simulink model "dpd_pa"  (Simulink 8.7)
settings: Solver=VariableStepDiscrete  StartTime=0.0  StopTime=hepta_dpd_pa_param.endTime  RelTol=1e-3
PreLoadFcn:
  | % Run the setup script when the model is opened
  | setup_dpd_pa;
InitFcn:
  | % Run the setup script again just before the
  | % model is run, so that any updates made
  | % after opening are applied.
  | setup_dpd_pa;
undefined symbols (not defined in the file or in its folder): AdvDSPBChannelOutDisplay, dpoly, dspba_ChannelInVis, dspba_ChannelOutVis, dspba_internal_get_channel_ports, evalAionMaskParam, hepta_dpd_pa_param, latency, value
libraries: DSPBAPrim x159, DSPBABase x6, DSPBAAvalonST x2, DSPBAUtilities x1
(part 2 of 2)

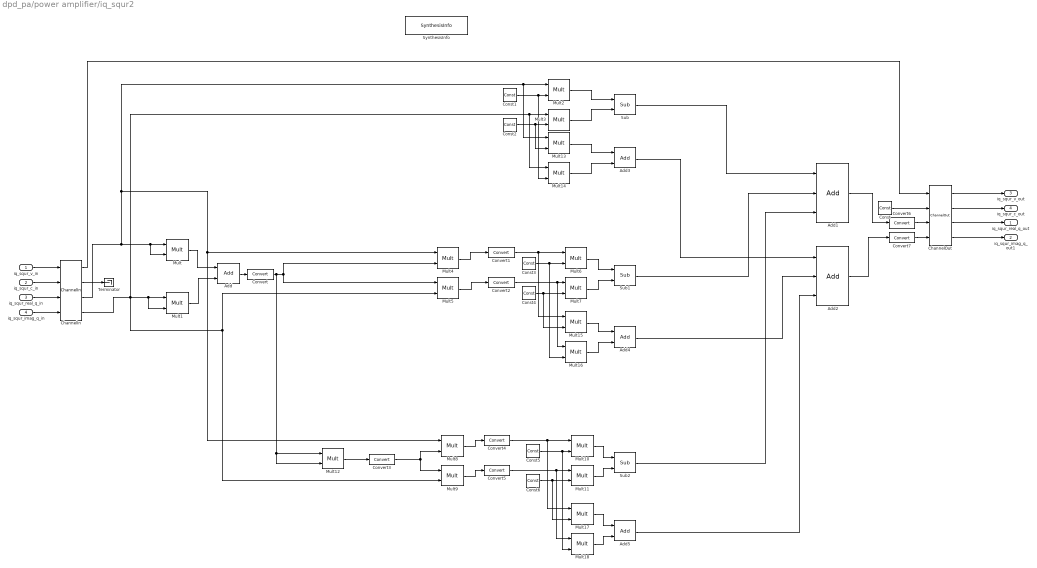
== system dpd_pa/power amplifier/iq_squr2 ==
  iq_squr_v_in : Inport
  iq_squr_c_in : Inport  Port=2
  iq_squr_real_q_in : Inport  Port=3
  iq_squr_imag_q_in : Inport  Port=4
  Add{,3..5} (4 alike) : DSPBAPrim/Add  primtype=add  nInputs=evalAionMaskParam(gcb,'value',1)  nOutputs=1  omode=Inherit via internal rule with word growth  otype=sfix(16)  scale=2^-15  rndmethod=Unbiased  factor=1  satmethod=Symmetric  shift_vec=[0 1 2 -1]  value=2  inPortNames=[' '; ' ';]  outPortNames=[' ']  dspbaimage=dspba_prim.jpg  text=fprintf('+');  style=Optimised  visibilities=1032+2^17+2^18+2^19  genFPC=off  floatRounding=correct  advOptions=[]  version=20130821
  Add1 : DSPBAPrim/Add  primtype=add  nInputs=evalAionMaskParam(gcb,'value',1)  nOutputs=1  omode=Inherit via internal rule with word growth  otype=sfix(16)  scale=2^-15  rndmethod=Unbiased  factor=1  satmethod=Symmetric  shift_vec=[0 1 2 -1]  value=3  inPortNames=[' '; ' ';]  outPortNames=[' ']  dspbaimage=dspba_prim.jpg  text=fprintf('+');  style=Optimised  visibilities=1032+2^17+2^18+2^19  genFPC=off  floatRounding=correct  advOptions=[]  version=20130821
  Add2 : DSPBAPrim/Add  primtype=add  nInputs=evalAionMaskParam(gcb,'value',1)  nOutputs=1  omode=Inherit via internal rule with word growth  otype=sfix(16)  scale=2^-15  rndmethod=Unbiased  factor=1  satmethod=Symmetric  shift_vec=[0 1 2 -1]  value=3  inPortNames=[' '; ' ';]  outPortNames=[' ']  dspbaimage=dspba_prim.jpg  text=fprintf('+');  style=Optimised  visibilities=1032+2^17+2^18+2^19  genFPC=off  floatRounding=correct  advOptions=[]  version=20130821
  ChannelIn : DSPBAPrim/ChannelIn  primtype=channelin  nInputs=dspba_internal_get_channel_ports(gcb)  nOutputs=dspba_internal_get_channel_ports(gcb)  omode=Inherit via internal rule  otype=sfix(16)  scale=2^-15  rndmethod=Unbiased  factor=1  satmethod=Symmetric  shift_vec=[0 1 2 -1]  value=2  inPortNames=['v'; 'c'; '0'; '1'; '2'; '3'; '4'; '5'; '6'; '7'; '8'; '9'; 'A'; 'B'; 'D'; 'E'; 'F'; 'G'; 'H'; 'I'; 'J'; 'K'; 'L'; 'M'; 'N'; 'O'; 'P'; 'Q'; 'R'; 'S'; 'T'; 'U'; 'W'; 'X'; 'Y'; 'Z']  outPortNames=['v'; 'c'; '0'; '1'; '2'; '3'; '4'; '5'; '6'; '7'; '8'; '9'; 'A'; 'B'; 'D'; 'E'; 'F'; 'G'; 'H'; 'I'; 'J'; 'K'; 'L'; 'M'; 'N'; 'O'; 'P'; 'Q'; 'R'; 'S'; 'T'; 'U'; 'W'; 'X'; 'Y'; 'Z']  dspbaimage=dspba_prim.jpg  text=fprintf('In');  style=Optimised  dataSignals=2  foldingEnabled=off  channels=1  sampleRate=200  packetBeginPresent=off  packetBeginEnabled=off  visibilities=dspba_ChannelInVis(gcb)  latencyCorrection=0  version=20141013
  ChannelOut : DSPBAPrim/ChannelOut  primtype=channelout  nInputs=dspba_internal_get_channel_ports(gcb)  nOutputs=dspba_internal_get_channel_ports(gcb)  omode=Inherit via internal rule  otype=sfix(16)  scale=2^-15  rndmethod=Unbiased  factor=1  satmethod=Symmetric  shift_vec=[0 1 2 -1]  value=2  inPortNames=['v'; 'c'; '0'; '1'; '2'; '3'; '4'; '5'; '6'; '7'; '8'; '9'; 'A'; 'B'; 'D'; 'E'; 'F'; 'G'; 'H'; 'I'; 'J'; 'K'; 'L'; 'M'; 'N'; 'O'; 'P'; 'Q'; 'R'; 'S'; 'T'; 'U'; 'W'; 'X'; 'Y'; 'Z']  outPortNames=['v'; 'c'; '0'; '1'; '2'; '3'; '4'; '5'; '6'; '7'; '8'; '9'; 'A'; 'B'; 'D'; 'E'; 'F'; 'G'; 'H'; 'I'; 'J'; 'K'; 'L'; 'M'; 'N'; 'O'; 'P'; 'Q'; 'R'; 'S'; 'T'; 'U'; 'W'; 'X'; 'Y'; 'Z']  dspbaimage=dspba_prim.jpg  text=fprintf('Out%s', AdvDSPBChannelOutDisplay(latency));  style=Optimised  dataSignals=2  foldingEnabled=off  channels=1  sampleRate=200  packetBeginPresent=off  packetBeginEnabled=off  visibilities=dspba_ChannelOutVis(gcb)  latency=15  latencyCorrection=0  version=20141013
  Const : DSPBAPrim/Const  primtype=const  nInputs=0  nOutputs=1  omode=Specify via dialog  otype=uint(8)  scale=0  rndmethod=Unbiased  factor=1  satmethod=Symmetric  shift_vec=[0 1 2 -1]  value=0  inPortNames=['+'; '+';]  outPortNames=[' ']  dspbaimage=dspba_prim.jpg  text=fprintf('%s', num2str(value));  style=Optimised  visibilities=8 + 1024  floatPrecision=float32_m23  version=20120820
  Const1 : DSPBAPrim/Const  primtype=const  nInputs=0  nOutputs=1  omode=Specify via dialog  otype=sfix(16)  scale=2^-15  rndmethod=Unbiased  factor=1  satmethod=Symmetric  shift_vec=[0 1 2 -1]  value=947  inPortNames=['+'; '+';]  outPortNames=[' ']  dspbaimage=dspba_prim.jpg  text=fprintf('%s', num2str(value));  style=Optimised  visibilities=8 + 1024  floatPrecision=float32_m23  version=20120820
  Const2 : DSPBAPrim/Const  primtype=const  nInputs=0  nOutputs=1  omode=Specify via dialog  otype=sfix(16)  scale=2^-15  rndmethod=Unbiased  factor=1  satmethod=Symmetric  shift_vec=[0 1 2 -1]  value=65359  inPortNames=['+'; '+';]  outPortNames=[' ']  dspbaimage=dspba_prim.jpg  text=fprintf('%s', num2str(value));  style=Optimised  visibilities=8 + 1024  floatPrecision=float32_m23  version=20120820
  Const3 : DSPBAPrim/Const  primtype=const  nInputs=0  nOutputs=1  omode=Specify via dialog  otype=sfix(16)  scale=2^-15  rndmethod=Unbiased  factor=1  satmethod=Symmetric  shift_vec=[0 1 2 -1]  value=63501  inPortNames=['+'; '+';]  outPortNames=[' ']  dspbaimage=dspba_prim.jpg  text=fprintf('%s', num2str(value));  style=Optimised  visibilities=8 + 1024  floatPrecision=float32_m23  version=20120820
  Const4 : DSPBAPrim/Const  primtype=const  nInputs=0  nOutputs=1  omode=Specify via dialog  otype=sfix(16)  scale=2^-15  rndmethod=Unbiased  factor=1  satmethod=Symmetric  shift_vec=[0 1 2 -1]  value=62482  inPortNames=['+'; '+';]  outPortNames=[' ']  dspbaimage=dspba_prim.jpg  text=fprintf('%s', num2str(value));  style=Optimised  visibilities=8 + 1024  floatPrecision=float32_m23  version=20120820
  Const5 : DSPBAPrim/Const  primtype=const  nInputs=0  nOutputs=1  omode=Specify via dialog  otype=sfix(16)  scale=2^-15  rndmethod=Unbiased  factor=1  satmethod=Symmetric  shift_vec=[0 1 2 -1]  value=4027  inPortNames=['+'; '+';]  outPortNames=[' ']  dspbaimage=dspba_prim.jpg  text=fprintf('%s', num2str(value));  style=Optimised  visibilities=8 + 1024  floatPrecision=float32_m23  version=20120820
  Const6 : DSPBAPrim/Const  primtype=const  nInputs=0  nOutputs=1  omode=Specify via dialog  otype=sfix(16)  scale=2^-15  rndmethod=Unbiased  factor=1  satmethod=Symmetric  shift_vec=[0 1 2 -1]  value=4941  inPortNames=['+'; '+';]  outPortNames=[' ']  dspbaimage=dspba_prim.jpg  text=fprintf('%s', num2str(value));  style=Optimised  visibilities=8 + 1024  floatPrecision=float32_m23  version=20120820
  Convert{,1..7} (8 alike) : DSPBAPrim/Convert  primtype=convert  nInputs=1  nOutputs=1  omode=Specify via dialog  otype=sfix(16)  scale=2^-15  rndmethod=Unbiased  factor=1  satmethod=None  shift_vec=[0 1 2 -1]  value=round([0:255]/17)  inPortNames=[' '; ' ';]  outPortNames=[' '; 'c']  dspbaimage=dspba_prim.jpg  text=fprintf('convert');  style=Optimised  visibilities=8+64+256+2^17  clipdetect=off  floatPrecision=float32_m23  advOptions=[]  version=20130211
  Mult{,1..18} (19 alike) : DSPBAPrim/Mult  primtype=mult  nInputs=2  nOutputs=1  omode=Inherit via internal rule  otype=sfix(16)  scale=2^-15  rndmethod=Unbiased  factor=1  satmethod=Symmetric  shift_vec=[0 1 2 -1]  value=0  inPortNames=[' '; ' ';]  outPortNames=[' ']  dspbaimage=dspba_prim.jpg  text=fprintf('X');  style=Optimised  visibilities=8+2^18+2^19  floatPrecision=float32_m23  floatRounding=correct  advOptions=[]  version=20130115
  Sub : DSPBAPrim/Sub  primtype=sub  nInputs=2  nOutputs=1  omode=Inherit via internal rule with word growth  otype=sfix(16)  scale=2^-15  rndmethod=Unbiased  factor=1  satmethod=Symmetric  shift_vec=[0 1 2 -1]  value=0  inPortNames=['+'; '-';]  outPortNames=[' ']  dspbaimage=dspba_prim.jpg  text=fprintf('-');  style=Optimised  visibilities=8+2^17+2^18  floatRounding=correct  advOptions=[]  version=20130115
  Sub1 : DSPBAPrim/Sub  primtype=sub  nInputs=2  nOutputs=1  omode=Inherit via internal rule with word growth  otype=sfix(16)  scale=2^-15  rndmethod=Unbiased  factor=1  satmethod=Symmetric  shift_vec=[0 1 2 -1]  value=0  inPortNames=['+'; '-';]  outPortNames=[' ']  dspbaimage=dspba_prim.jpg  text=fprintf('-');  style=Optimised  visibilities=8+2^17+2^18  floatRounding=correct  advOptions=[]  version=20130115
  Sub2 : DSPBAPrim/Sub  primtype=sub  nInputs=2  nOutputs=1  omode=Inherit via internal rule with word growth  otype=sfix(16)  scale=2^-15  rndmethod=Unbiased  factor=1  satmethod=Symmetric  shift_vec=[0 1 2 -1]  value=0  inPortNames=['+'; '-';]  outPortNames=[' ']  dspbaimage=dspba_prim.jpg  text=fprintf('-');  style=Optimised  visibilities=8+2^17+2^18  floatRounding=correct  advOptions=[]  version=20130115
  SynthesisInfo : DSPBAPrim/SynthesisInfo  primtype=synthinfo  nInputs=0  nOutputs=0  omode=Inherit via internal rule  otype=sfix(16)  scale=2^-15  rndmethod=Truncate  factor=1  satmethod=Symmetric  shift_vec=[0 1 2 -1]  value=99  inPortNames=[' '; ' ';]  outPortNames=[' ']  dspbaimage=dspba_prim_ctrl.jpg  text=fprintf('Style=%s', style);  style=Scheduled  visibilities=2^15+2^17+2^18+2^19  constraintInUse=off  constraintRelation=>  constraintLimit=2  bitAccurate=off  version=20150220
  Terminator : Terminator
  iq_squr_real_q_out : Outport
  iq_squr_imag_q_out1 : Outport  Port=2
  iq_squr_v_out : Outport  Port=3
  iq_squr_c_out : Outport  Port=4
  wires:
  Mult/1 -> Add/1
  Mult1/1 -> Add/2
  iq_squr_imag_q_in/1 -> ChannelIn/4
  iq_squr_real_q_in/1 -> ChannelIn/3
  ChannelOut/3 -> iq_squr_real_q_out/1
  ChannelOut/1 -> iq_squr_v_out/1
  ChannelOut/2 -> iq_squr_c_out/1
  iq_squr_v_in/1 -> ChannelIn/1
  iq_squr_c_in/1 -> ChannelIn/2
  ChannelIn/2 -> Terminator/1
  ChannelIn/3 -> Mult13/1, Mult2/1, Mult8/1, Mult4/1, Mult/2, Mult/1
  ChannelIn/4 -> Mult14/1, Mult3/1, Mult5/2, Mult9/2, Mult1/2, Mult1/1
  Const/1 -> ChannelOut/2
  Add/1 -> Convert/1
  Const3/1 -> Mult16/2, Mult6/2
  Const4/1 -> Mult15/2, Mult7/2
  Mult4/1 -> Convert1/1
  Mult5/1 -> Convert2/1
  Const5/1 -> Mult18/2, Mult10/2
  Const6/1 -> Mult17/2, Mult11/2
  Mult8/1 -> Convert4/1
  Mult9/1 -> Convert5/1
  Mult12/1 -> Convert3/1
  Convert/1 -> Mult12/2, Mult12/1, Mult5/1, Mult4/2
  Convert1/1 -> Mult15/1, Mult6/1
  Convert2/1 -> Mult16/1, Mult7/1
  Convert3/1 -> Mult9/1, Mult8/2
  Convert4/1 -> Mult17/1, Mult10/1
  Convert5/1 -> Mult18/1, Mult11/1
  Add1/1 -> Convert6/1
  Add2/1 -> Convert7/1
  ChannelIn/1 -> ChannelOut/1
  Convert6/1 -> ChannelOut/3
  Convert7/1 -> ChannelOut/4
  ChannelOut/4 -> iq_squr_imag_q_out1/1
  Const1/1 -> Mult14/2, Mult2/2
  Const2/1 -> Mult13/2, Mult3/2
  Mult2/1 -> Sub/1
  Mult3/1 -> Sub/2
  Mult13/1 -> Add3/1
  Mult14/1 -> Add3/2
  Sub/1 -> Add1/1
  Add3/1 -> Add2/1
  Mult6/1 -> Sub1/1
  Mult7/1 -> Sub1/2
  Mult15/1 -> Add4/1
  Mult16/1 -> Add4/2
  Sub1/1 -> Add1/2
  Add4/1 -> Add2/2
  Mult10/1 -> Sub2/1
  Mult11/1 -> Sub2/2
  Mult17/1 -> Add5/1
  Mult18/1 -> Add5/2
  Add5/1 -> Add2/3
  Sub2/1 -> Add1/3
